simulink model "save_data"  (R2019b)
settings: Solver=FixedStepDiscrete  StartTime=0.0  StopTime=Inf  FixedStep=1/200  RelTol=1e-3  EnableMultiTasking=on
libraries: xpcrtudplib x1, xpcutilitieslib x1
settings Model: Creator=student  LastModifiedBy=student
settings DataIOCC: LimitDataPoints=on  SaveFormat=Array  ReturnWorkspaceOutputs=off
settings OptimizationCC: LifeSpan=inf
settings DebuggingCC: SolverPrmCheckMsg=warning  SFUnexpectedBacktrackingDiag=warning  SFNoUnconditionalDefaultTransitionDiag=warning  SFExecutionAtInitializationDiag=none  ArithmeticOperatorsInVariantConditions=warning
settings HardwareCC: ProdBitPerPointer=32  ProdBitPerSizeT=32  ProdBitPerPtrDiffT=32  ProdLargestAtomicFloat=None  ProdIntDivRoundTo=Undefined  ProdEndianess=Unspecified  ProdWordSize=32  ProdHWDeviceType=32-bit Generic
settings ModelReferenceCC: PropagateSignalLabelsOutOfModel=off
settings SFSimCC: SimUseLocalCustomCode=off  CustomCodeUndefinedFunction=UseInterfaceOnly
settings RTWCC: RTWUseLocalCustomCode=off
settings CodeAppCC: StateflowObjectComments=on
settings GRTTargetCC: TargetLangStandard=C89/C90 (ANSI)  GeneratePreprocessorConditionals=Disable all
settings ConfigComp: CovMetricSettings=dw  CovHtmlReporting=on  CovSaveCumulativeToWorkspaceVar=on  CovSaveSingleToWorkspaceVar=on  CovExternalEMLEnable=off  CovSFcnEnable=off

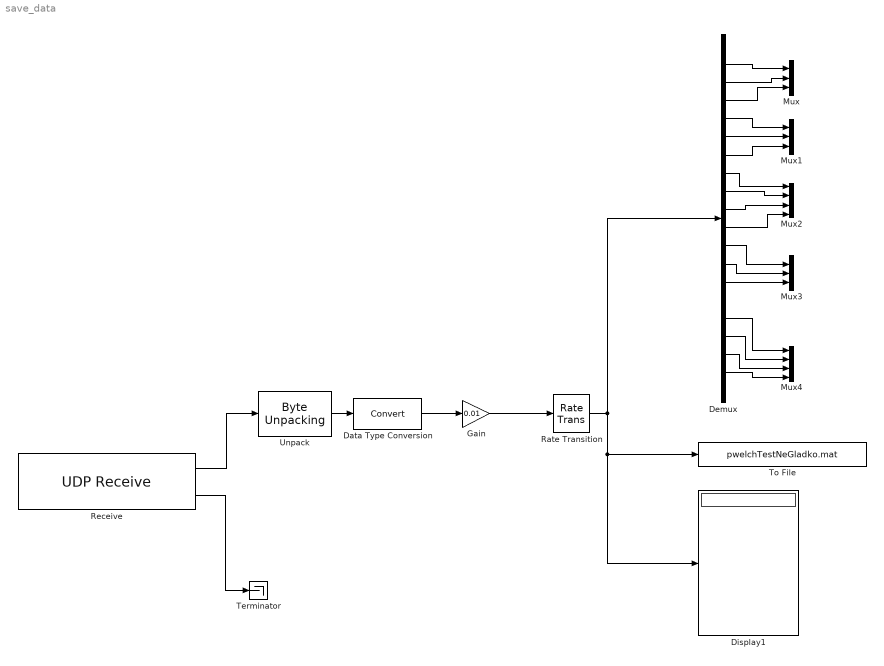
== system save_data ==
  Data Type Conversion : DataTypeConversion
  Demux : Demux  Outputs=18
  Display1 : Display
  Gain : Gain  Gain=0.01
  Mux : Mux  Inputs=3
  Mux1 : Mux  Inputs=3
  Mux2 : Mux
  Mux3 : Mux  Inputs=3
  Mux4 : Mux
  Rate Transition : RateTransition
  "Receive " : xpcrtudplib/UDP Receive  ipAddressVal=Use host-target connection  localPort=25008  rcvWidth=328  rcvFmAny=off  fmAddress=192.168.65.241  rcvMulticast=off  multicastAddress={}  maxUDPQueue=8  sampleTime=0.01
      settings: SourceProductName=Simulink Real-Time
  Terminator : Terminator
  To File : ToFile  Filename=pwelchTestNeGladko.mat
  "Unpack " : xpcutilitieslib/Byte Unpacking   MaskUnpackedDataTypes={'single'}  MaskUnpackedDataSizes={[82]}  MaskAlignment=1
      settings: SourceProductName=Simulink Real-Time  SourceProductBaseCode=XP
  wires:
  "Receive "/2 -> Terminator/1
  "Receive "/1 -> "Unpack "/1
  Rate Transition/1 -> Display1/1, To File/1, Demux/1
  "Unpack "/1 -> Data Type Conversion/1
  Data Type Conversion/1 -> Gain/1
  Gain/1 -> Rate Transition/1
  Demux/1 -> Mux/1
  Demux/2 -> Mux/2
  Demux/3 -> Mux/3
  Demux/4 -> Mux1/1
  Demux/5 -> Mux1/2
  Demux/6 -> Mux1/3
  Demux/7 -> Mux2/1
  Demux/8 -> Mux2/2
  Demux/9 -> Mux2/3
  Demux/10 -> Mux2/4
  Demux/11 -> Mux3/1
  Demux/12 -> Mux3/2
  Demux/13 -> Mux3/3
  Demux/18 -> Mux4/4
  Demux/17 -> Mux4/3
  Demux/16 -> Mux4/2
  Demux/15 -> Mux4/1
